simulink model "TriggeredSystem"  (R2016a)
settings: Solver=FixedStepDiscrete  StartTime=0.0  StopTime=0.03  RelTol=1e-3
settings Model: Creator=hp  LastModifiedBy=hp
settings OptimizationCC: DefaultParameterBehavior=Inlined  OptimizeModelRefInitCode=on  LifeSpan=1
settings DebuggingCC: UnderspecifiedInitializationDetection=Classic  MergeDetectMultiDrivingBlocksExec=none
settings ModelReferenceCC: PropagateSignalLabelsOutOfModel=off
settings RTWCC: SystemTargetFile=ert.tlc  GenCodeOnly=on  TemplateMakefile=ert_default_tmf  GenerateReport=on  IncludeHyperlinkInReport=on  LaunchReport=on  GenerateTraceInfo=on  GenerateTraceReport=on  GenerateTraceReportSl=on  GenerateTraceReportSf=on  GenerateTraceReportEml=on
settings CodeAppCC: ForceParamTrailComments=on  IgnoreCustomStorageClasses=off  OperatorAnnotations=on  SimulinkDataObjDesc=on  SFDataObjDesc=on  MATLABFcnDesc=on  InsertBlockDesc=on  MATLABSourceComments=on
settings ERTTargetCC: GenerateSampleERTMain=on  InlinedParameterPlacement=NonHierarchical  ERTCustomFileTemplate=example_file_process.tlc

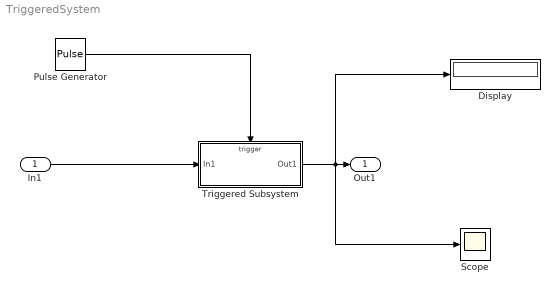
== system TriggeredSystem ==
  In1 : Inport
  Display : Display
  Pulse Generator : DiscretePulseGenerator  PulseType=Time based  Period=0.005  PulseWidth=50
  Scope : Scope
  Triggered Subsystem : Subsystem  TreatAsAtomicUnit=on
  Out1 : Outport
  wires:
  Pulse Generator/1 -> Triggered Subsystem/Trigger
  Triggered Subsystem/1(Out1) -> Scope/1, Display/1, Out1/1
  In1/1 -> Triggered Subsystem/1(In1)

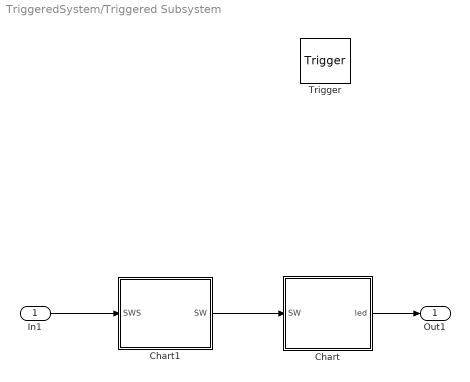
== system TriggeredSystem/Triggered Subsystem ==
  In1 : Inport
  Trigger : TriggerPort  VariantControl=Variant
  Chart : Stateflow chart  TreatAsAtomicUnit=on
  Chart1 : Stateflow chart  TreatAsAtomicUnit=on
  Out1 : Outport
  wires:
  Chart/1(led) -> Out1/1
  In1/1 -> Chart1/1(SWS)
  Chart1/1(SW) -> Chart/1(SW)

== stateflow chart TriggeredSystem/Triggered Subsystem/Chart1 ==
  (default) -> (junction 29)
  (junction 29) -> (junction 30) [order 1] : [SWS == 1]
  (junction 29) -> (junction 31) [order 2] : {SW = 0;}
  (junction 30) -> (junction 32) : {SW = 1;}
  (junction 32) -> (junction 31)
  (junction 31) -> (junction 33)
  data: SWS input; SW output uint8

== stateflow chart TriggeredSystem/Triggered Subsystem/Chart ==
  (default) -> (junction 9)
  (junction 9) -> (junction 10) [order 1] : [SW == 1]
  (junction 9) -> (junction 11) [order 2] : {led = uint8(0);}
  (junction 10) -> (junction 12) : {led = uint8(1);}
  (junction 12) -> (junction 11)
  (junction 11) -> (junction 13)
  data: led output uint8; SW input uint8
